simulink model "IEEE14_case"  (R2024b)
settings: Solver=FixedStepAuto  StartTime=0  StopTime=2  FixedStep=1e-7  RelTol=1e-3
values from neighbouring files (symbols this model uses):
  GFL_15_Bva = 0.009    [IEEE14_parameters.m]
  GFL_15_C_bus_pu = 7.179419    [IEEE14_parameters.m]
  GFL_15_f0 = 60    [IEEE14_parameters.m]
  GFL_15_I_id = 691.26967    [IEEE14_parameters.m]
  GFL_15_I_iq = 691.26967    [IEEE14_parameters.m]
  GFL_15_I_od = 45.2207    [IEEE14_parameters.m]
  GFL_15_I_oq = 45.2207    [IEEE14_parameters.m]
  GFL_15_I_pll = 0.78    [IEEE14_parameters.m]
  GFL_15_Kdi = 0.09    [IEEE14_parameters.m]
  GFL_15_Kdo = 0.9    [IEEE14_parameters.m]
  GFL_15_Kqi = 0.09    [IEEE14_parameters.m]
  GFL_15_Kqo = 0.9    [IEEE14_parameters.m]
  GFL_15_Lg_pu = 0.631447    [IEEE14_parameters.m]
  GFL_15_mode = 1    [IEEE14_parameters.m]
  GFL_15_P_id = 3.7166    [IEEE14_parameters.m]
  GFL_15_P_iq = 3.7166    [IEEE14_parameters.m]
  GFL_15_P_od = 0.4798    [IEEE14_parameters.m]
  GFL_15_P_oq = 0.4798    [IEEE14_parameters.m]
  GFL_15_P_pll = 290.42    [IEEE14_parameters.m]
  GFL_15_Qe_ref = 0.2    [IEEE14_parameters.m]
  GFL_15_Rg_pu = 0.024016    [IEEE14_parameters.m]
  GFL_15_Sbase = 1.000000e+4    (= 10000)    [IEEE14_parameters.m]
  GFL_15_Tdi = 0.01    [IEEE14_parameters.m]
  GFL_15_Tdo = 0.2    [IEEE14_parameters.m]
  GFL_15_Tqi = 0.01    [IEEE14_parameters.m]
  GFL_15_Tqo = 0.2    [IEEE14_parameters.m]
  GFL_15_Vbase = 380    [IEEE14_parameters.m]
  GFL_15_Vdc_ref = 1.011475    [IEEE14_parameters.m]
  GFL_15_Vdcbase = 700    [IEEE14_parameters.m]
  GFL_15_vq_ref = 0    [IEEE14_parameters.m]
  GFL_16_Bva = 0.002    [IEEE14_parameters.m]
  GFL_16_C_bus_pu = 7.179419    [IEEE14_parameters.m]
  GFL_16_f0 = 60    [IEEE14_parameters.m]
  GFL_16_I_id = 691.26967    [IEEE14_parameters.m]
  GFL_16_I_iq = 691.26967    [IEEE14_parameters.m]
  GFL_16_I_od = 45.2207    [IEEE14_parameters.m]
  GFL_16_I_oq = 45.2207    [IEEE14_parameters.m]
  GFL_16_I_pll = 0.78    [IEEE14_parameters.m]
  GFL_16_Kdi = 0.05    [IEEE14_parameters.m]
  GFL_16_Kdo = 0.5    [IEEE14_parameters.m]
  GFL_16_Kqi = 0.05    [IEEE14_parameters.m]
  GFL_16_Kqo = 0.5    [IEEE14_parameters.m]
  GFL_16_Lg_pu = 0.631447    [IEEE14_parameters.m]
  GFL_16_mode = 1    [IEEE14_parameters.m]
  GFL_16_P_id = 3.7166    [IEEE14_parameters.m]
  GFL_16_P_iq = 3.7166    [IEEE14_parameters.m]
  GFL_16_P_od = 0.4798    [IEEE14_parameters.m]
  GFL_16_P_oq = 0.4798    [IEEE14_parameters.m]
  GFL_16_P_pll = 290.42    [IEEE14_parameters.m]
  GFL_16_Qe_ref = 0.2    [IEEE14_parameters.m]
  GFL_16_Rg_pu = 0.024016    [IEEE14_parameters.m]
  GFL_16_Sbase = 1.000000e+4    (= 10000)    [IEEE14_parameters.m]
  GFL_16_Tdi = 0.01    [IEEE14_parameters.m]
  GFL_16_Tdo = 0.2    [IEEE14_parameters.m]
  GFL_16_Tqi = 0.01    [IEEE14_parameters.m]
  GFL_16_Tqo = 0.2    [IEEE14_parameters.m]
  GFL_16_Vbase = 380    [IEEE14_parameters.m]
  GFL_16_Vdc_ref = 1.01144    [IEEE14_parameters.m]
  GFL_16_Vdcbase = 700    [IEEE14_parameters.m]
  GFL_16_vq_ref = 0    [IEEE14_parameters.m]
  GFL_17_Bva = 0.002    [IEEE14_parameters.m]
  GFL_17_C_bus_pu = 7.179419    [IEEE14_parameters.m]
  GFL_17_f0 = 60    [IEEE14_parameters.m]
  GFL_17_I_id = 691.26967    [IEEE14_parameters.m]
  GFL_17_I_iq = 691.26967    [IEEE14_parameters.m]
  GFL_17_I_od = 45.2207    [IEEE14_parameters.m]
  GFL_17_I_oq = 45.2207    [IEEE14_parameters.m]
  GFL_17_I_pll = 0.78    [IEEE14_parameters.m]
  GFL_17_Kdi = 0.05    [IEEE14_parameters.m]
  GFL_17_Kdo = 0.5    [IEEE14_parameters.m]
  GFL_17_Kqi = 0.05    [IEEE14_parameters.m]
  GFL_17_Kqo = 0.5    [IEEE14_parameters.m]
  GFL_17_Lg_pu = 0.631447    [IEEE14_parameters.m]
  GFL_17_mode = 1    [IEEE14_parameters.m]
  GFL_17_P_id = 3.7166    [IEEE14_parameters.m]
  GFL_17_P_iq = 3.7166    [IEEE14_parameters.m]
  GFL_17_P_od = 0.4798    [IEEE14_parameters.m]
  GFL_17_P_oq = 0.4798    [IEEE14_parameters.m]
  GFL_17_P_pll = 290.42    [IEEE14_parameters.m]
  GFL_17_Qe_ref = 0.2    [IEEE14_parameters.m]
  GFL_17_Rg_pu = 0.024016    [IEEE14_parameters.m]
  GFL_17_Sbase = 1.000000e+4    (= 10000)    [IEEE14_parameters.m]
  GFL_17_Tdi = 0.01    [IEEE14_parameters.m]
  GFL_17_Tdo = 0.2    [IEEE14_parameters.m]
  GFL_17_Tqi = 0.01    [IEEE14_parameters.m]
  GFL_17_Tqo = 0.2    [IEEE14_parameters.m]
  GFL_17_Vbase = 380    [IEEE14_parameters.m]
  GFL_17_Vdc_ref = 1.011632    [IEEE14_parameters.m]
  GFL_17_Vdcbase = 700    [IEEE14_parameters.m]
  GFL_17_vq_ref = 0    [IEEE14_parameters.m]
  GFL_18_Bva = 0.002    [IEEE14_parameters.m]
  GFL_18_C_bus_pu = 7.179419    [IEEE14_parameters.m]
  GFL_18_f0 = 60    [IEEE14_parameters.m]
  GFL_18_I_id = 691.26967    [IEEE14_parameters.m]
  GFL_18_I_iq = 691.26967    [IEEE14_parameters.m]
  GFL_18_I_od = 45.2207    [IEEE14_parameters.m]
  GFL_18_I_oq = 45.2207    [IEEE14_parameters.m]
  GFL_18_I_pll = 0.78    [IEEE14_parameters.m]
  GFL_18_Kdi = 0.05    [IEEE14_parameters.m]
  GFL_18_Kdo = 0.5    [IEEE14_parameters.m]
  GFL_18_Kqi = 0.05    [IEEE14_parameters.m]
  GFL_18_Kqo = 0.5    [IEEE14_parameters.m]
  GFL_18_Lg_pu = 0.631447    [IEEE14_parameters.m]
  GFL_18_mode = 1    [IEEE14_parameters.m]
  GFL_18_P_id = 3.7166    [IEEE14_parameters.m]
  GFL_18_P_iq = 3.7166    [IEEE14_parameters.m]
  GFL_18_P_od = 0.4798    [IEEE14_parameters.m]
  GFL_18_P_oq = 0.4798    [IEEE14_parameters.m]
  GFL_18_P_pll = 290.42    [IEEE14_parameters.m]
  GFL_18_Qe_ref = 0.2    [IEEE14_parameters.m]
  GFL_18_Rg_pu = 0.024016    [IEEE14_parameters.m]
  GFL_18_Sbase = 1.000000e+4    (= 10000)    [IEEE14_parameters.m]
  GFL_18_Tdi = 0.01    [IEEE14_parameters.m]
  GFL_18_Tdo = 0.2    [IEEE14_parameters.m]
  GFL_18_Tqi = 0.01    [IEEE14_parameters.m]
  GFL_18_Tqo = 0.2    [IEEE14_parameters.m]
  GFL_18_Vbase = 380    [IEEE14_parameters.m]
  GFL_18_Vdc_ref = 1.011572    [IEEE14_parameters.m]
  GFL_18_Vdcbase = 700    [IEEE14_parameters.m]
  GFL_18_vq_ref = 0    [IEEE14_parameters.m]
  ... (+180 more)
(part 14 of 25)

== system IEEE14_case/GFL_18/d_Phi_gb_GFL_18_block ==
  note: d_Phi_gb_GFL_18 in case14gfl
      | $I_{\mathrm{id}}\,\left(\mathrm{Idv}_{\mathrm{GFL},18}+\Phi _{\mathrm{ga},\mathrm{GFL},18}-i_{\mathrm{gd},\mathrm{GFL},18}+P_{\mathrm{od}}\,\left(V_{\mathrm{dc},\mathrm{GFL},18}-\mathrm{Vdcbase}\,\mathrm{Vdc}_{\mathrm{ref}}\right)-\mathrm{Bva}\,\mathrm{Vbase}\,\left(v_{d,\mathrm{GFL},18}\,\cos\left(\theta _{\mathrm{pll},\mathrm{GFL},18}\right)-v_{q,\mathrm{GFL},18}\,\sin\left(\theta _{\mathrm{pll},\mathrm{GFL},18}\right)\right)\right)$
      | Automatically generated on 2025-10-09 21:37:49 .
  Input_v_d_GFL_18_d4937 : Inport
  State_theta_pll_GFL_18_76645 : Inport  Port=2
  Input_v_q_GFL_18_3c3a2 : Inport  Port=3
  State_theta_pll_GFL_18_60c54 : Inport  Port=4
  State_Idv_GFL_18_7a112 : Inport  Port=5
  State_V_dc_GFL_18_6f965 : Inport  Port=6
  State_Phi_ga_GFL_18_0803b : Inport  Port=7
  State_i_gd_GFL_18_25876 : Inport  Port=8
  Add_04fac : Sum
  Add_50ceb : Sum
  Add_6d765 : Sum
  Constant_-1_9318c : Constant  Value=-1
  Constant_Bva_df253 : Constant  Value=Bva
  Constant_I_id_6af81 : Constant  Value=I_id
  Constant_P_od_38045 : Constant  Value=P_od
  Constant_Vbase_96544 : Constant  Value=Vbase
  Constant_Vdc_ref_6e116 : Constant  Value=Vdc_ref
  Constant_Vdcbase_8f6c7 : Constant  Value=Vdcbase
  MathFunc_cos_a7f41 : Trigonometry  Operator=cos
  MathFunc_sin_0412c : Trigonometry
  Product_07db6 : Product
  Product_24552 : Product
  Product_2c113 : Product
  Product_61e81 : Product
  Product_6af82 : Product
  Product_85d52 : Product
  Product_860c9 : Product
  Product_f2f88 : Product
  Subtract_3a44e : Sum  Inputs=+-
  Subtract_78130 : Sum  Inputs=+-
  Subtract_7a8e3 : Sum  Inputs=+-
  Blockout_d_Phi_gb_GFL_18_4adfd : Outport
  wires:
  State_theta_pll_GFL_18_76645/1 -> MathFunc_cos_a7f41/1
  MathFunc_cos_a7f41/1 -> Product_61e81/2
  State_theta_pll_GFL_18_60c54/1 -> MathFunc_sin_0412c/1
  Constant_Bva_df253/1 -> Product_24552/2
  MathFunc_sin_0412c/1 -> Product_2c113/2
  Constant_-1_9318c/1 -> Product_24552/1
  State_i_gd_GFL_18_25876/1 -> Subtract_7a8e3/2
  Product_61e81/1 -> Subtract_78130/1
  Input_v_d_GFL_18_d4937/1 -> Product_61e81/1
  Input_v_q_GFL_18_3c3a2/1 -> Product_2c113/1
  Product_24552/1 -> Product_85d52/1
  Constant_Vbase_96544/1 -> Product_85d52/2
  Product_2c113/1 -> Subtract_78130/2
  Constant_I_id_6af81/1 -> Product_f2f88/1
  Product_6af82/1 -> Subtract_3a44e/2
  Constant_Vdc_ref_6e116/1 -> Product_6af82/1
  Constant_Vdcbase_8f6c7/1 -> Product_6af82/2
  State_Idv_GFL_18_7a112/1 -> Add_04fac/2
  Product_85d52/1 -> Product_07db6/1
  State_Phi_ga_GFL_18_0803b/1 -> Add_50ceb/2
  Subtract_78130/1 -> Product_07db6/2
  Subtract_3a44e/1 -> Product_860c9/2
  State_V_dc_GFL_18_6f965/1 -> Subtract_3a44e/1
  Product_07db6/1 -> Add_04fac/1
  Constant_P_od_38045/1 -> Product_860c9/1
  Add_04fac/1 -> Add_6d765/1
  Product_860c9/1 -> Add_6d765/2
  Add_6d765/1 -> Add_50ceb/1
  Add_50ceb/1 -> Subtract_7a8e3/1
  Product_f2f88/1 -> Blockout_d_Phi_gb_GFL_18_4adfd/1
  Subtract_7a8e3/1 -> Product_f2f88/2

== system IEEE14_case/GFL_18/d_Phi_gc_GFL_18_block ==
  note: d_Phi_gc_GFL_18 in case14gfl
      | $-I_{\mathrm{oq}}\,\left(\mathrm{Qe}_{\mathrm{ref}}\,\mathrm{Sbase}+1.73205080756888\,\mathrm{Vbase}\,i_{\mathrm{gd},\mathrm{GFL},18}\,\left(v_{q,\mathrm{GFL},18}\,\cos\left(\theta _{\mathrm{pll},\mathrm{GFL},18}\right)+v_{d,\mathrm{GFL},18}\,\sin\left(\theta _{\mathrm{pll},\mathrm{GFL},18}\right)\right)+1.73205080756888\,\mathrm{Vbase}\,i_{\mathrm{gq},\mathrm{GFL},18}\,\left(v_{d,\mathrm{GFL},18}\,\cos\left(\theta _{\mathrm{pll},\mathrm{GFL},18}\right)-v_{q,\mathrm{GFL},18}\,\sin\left(\theta _{\mathrm{pll},\mathrm{GFL},18}\right)\right)\right)$
      | Automatically generated on 2025-10-09 21:37:52 .
  State_i_gd_GFL_18_5899c : Inport
  Input_v_d_GFL_18_02ef3 : Inport  Port=2
  State_theta_pll_GFL_18_ce778 : Inport  Port=3
  Input_v_q_GFL_18_ef739 : Inport  Port=4
  State_theta_pll_GFL_18_3fc4b : Inport  Port=5
  State_i_gq_GFL_18_622c8 : Inport  Port=6
  Input_v_d_GFL_18_79bfc : Inport  Port=7
  State_theta_pll_GFL_18_d8932 : Inport  Port=8
  Input_v_q_GFL_18_a00d2 : Inport  Port=9
  State_theta_pll_GFL_18_57f3c : Inport  Port=10
  Add_6d69b : Sum
  Constant_-1_98670 : Constant  Value=-1
  Constant_1.73205080756888_14d38 : Constant  Value=1.73205080756888
  Constant_1.73205080756888_ac93c : Constant  Value=1.73205080756888
  Constant_I_oq_ead3f : Constant  Value=I_oq
  Constant_Qe_ref_2b81e : Constant  Value=Qe_ref
  Constant_Sbase_95d0b : Constant  Value=Sbase
  Constant_Vbase_70aa7 : Constant  Value=Vbase
  Constant_Vbase_7f599 : Constant  Value=Vbase
  MathFunc_cos_52954 : Trigonometry  Operator=cos
  MathFunc_cos_58d6c : Trigonometry  Operator=cos
  MathFunc_sin_00400 : Trigonometry
  MathFunc_sin_37ab1 : Trigonometry
  Product_0c2bb : Product
  Product_12f9b : Product
  Product_31362 : Product
  Product_3452c : Product
  Product_405b1 : Product
  Product_472e4 : Product
  Product_90b14 : Product
  Product_9a0a3 : Product
  Product_a7161 : Product
  Product_ae793 : Product
  Product_e9756 : Product
  Product_eaf4c : Product
  Product_f56c9 : Product
  Subtract_514a8 : Sum  Inputs=+-
  Subtract_9ec50 : Sum  Inputs=+-
  Subtract_a8992 : Sum  Inputs=+-
  Blockout_d_Phi_gc_GFL_18_de35a : Outport
  wires:
  State_theta_pll_GFL_18_ce778/1 -> MathFunc_sin_00400/1
  MathFunc_sin_00400/1 -> Product_9a0a3/2
  Product_f56c9/1 -> Product_ae793/1
  Constant_Qe_ref_2b81e/1 -> Product_e9756/2
  Constant_Vbase_70aa7/1 -> Product_90b14/2
  State_theta_pll_GFL_18_3fc4b/1 -> MathFunc_cos_52954/1
  Constant_1.73205080756888_14d38/1 -> Product_90b14/1
  Product_e9756/1 -> Product_3452c/1
  Constant_-1_98670/1 -> Product_e9756/1
  Input_v_d_GFL_18_02ef3/1 -> Product_9a0a3/1
  Input_v_q_GFL_18_ef739/1 -> Product_eaf4c/1
  MathFunc_cos_52954/1 -> Product_eaf4c/2
  State_theta_pll_GFL_18_d8932/1 -> MathFunc_cos_58d6c/1
  State_theta_pll_GFL_18_57f3c/1 -> MathFunc_sin_37ab1/1
  Constant_Vbase_7f599/1 -> Product_0c2bb/2
  Product_90b14/1 -> Product_31362/1
  Product_0c2bb/1 -> Product_f56c9/1
  State_i_gd_GFL_18_5899c/1 -> Product_31362/2
  Product_9a0a3/1 -> Add_6d69b/1
  Product_eaf4c/1 -> Add_6d69b/2
  Constant_1.73205080756888_ac93c/1 -> Product_0c2bb/1
  Input_v_d_GFL_18_79bfc/1 -> Product_12f9b/1
  MathFunc_cos_58d6c/1 -> Product_12f9b/2
  Product_472e4/1 -> Subtract_514a8/2
  Input_v_q_GFL_18_a00d2/1 -> Product_472e4/1
  MathFunc_sin_37ab1/1 -> Product_472e4/2
  Constant_Sbase_95d0b/1 -> Product_3452c/2
  Product_31362/1 -> Product_405b1/1
  Add_6d69b/1 -> Product_405b1/2
  Constant_I_oq_ead3f/1 -> Product_a7161/1
  State_i_gq_GFL_18_622c8/1 -> Product_f56c9/2
  Product_12f9b/1 -> Subtract_514a8/1
  Product_3452c/1 -> Subtract_9ec50/1
  Product_405b1/1 -> Subtract_9ec50/2
  Subtract_514a8/1 -> Product_ae793/2
  Product_ae793/1 -> Subtract_a8992/2
  Subtract_9ec50/1 -> Subtract_a8992/1
  Subtract_a8992/1 -> Product_a7161/2
  Product_a7161/1 -> Blockout_d_Phi_gc_GFL_18_de35a/1

== system IEEE14_case/GFL_18/d_Phi_gd_GFL_18_block ==
  note: d_Phi_gd_GFL_18 in case14gfl
      | $I_{\mathrm{iq}}\,\left(\mathrm{Iqv}_{\mathrm{GFL},18}+\Phi _{\mathrm{gc},\mathrm{GFL},18}-i_{\mathrm{gq},\mathrm{GFL},18}-P_{\mathrm{oq}}\,\left(\mathrm{Qe}_{\mathrm{ref}}\,\mathrm{Sbase}+1.73205080756888\,\mathrm{Vbase}\,i_{\mathrm{gd},\mathrm{GFL},18}\,\left(v_{q,\mathrm{GFL},18}\,\cos\left(\theta _{\mathrm{pll},\mathrm{GFL},18}\right)+v_{d,\mathrm{GFL},18}\,\sin\left(\theta _{\mathrm{pll},\mathrm{GFL},18}\right)\right)+1.73205080756888\,\mathrm{Vbase}\,i_{\mathrm{gq},\mathrm{GFL},18}\,\left(v_{d,\mathrm{GFL},18}\,\cos\left(\theta _{\mathrm{pll},\mathrm{GFL},18}\right)-v_{q,\mathrm{GFL},18}\,\sin\left(\theta _{\mathrm{pll},\mathrm{GFL},18}\right)\right)\right)+\mathrm{Bva}\,\mathrm{Vbase}\,\left(v_{q,\mathrm{GFL},18}\,\cos\left(\theta _{\mathrm{pll},\mathrm{GFL},18}\right)+v_{d,\mathrm{GFL},18}\,\sin\left(\theta _{\mathrm{pll},\mathrm{GFL},18}\right)\right)\right)$
      | Automatically generated on 2025-10-09 21:37:55 .
  Input_v_d_GFL_18_11d9f : Inport
  State_theta_pll_GFL_18_6022b : Inport  Port=2
  Input_v_q_GFL_18_3c803 : Inport  Port=3
  State_theta_pll_GFL_18_7f5d8 : Inport  Port=4
  State_Iqv_GFL_18_70c7a : Inport  Port=5
  State_i_gd_GFL_18_2dd77 : Inport  Port=6
  Input_v_d_GFL_18_27679 : Inport  Port=7
  State_theta_pll_GFL_18_40df2 : Inport  Port=8
  Input_v_q_GFL_18_95c1e : Inport  Port=9
  State_theta_pll_GFL_18_8d0fd : Inport  Port=10
  State_i_gq_GFL_18_21998 : Inport  Port=11
  Input_v_d_GFL_18_ab6ff : Inport  Port=12
  State_theta_pll_GFL_18_77a50 : Inport  Port=13
  Input_v_q_GFL_18_9cd88 : Inport  Port=14
  State_theta_pll_GFL_18_ec069 : Inport  Port=15
  State_Phi_gc_GFL_18_ff2c0 : Inport  Port=16
  State_i_gq_GFL_18_464a8 : Inport  Port=17
  Add_0e427 : Sum
  Add_719c3 : Sum
  Add_c28f7 : Sum
  Add_c4a0d : Sum
  Add_f7ea7 : Sum
  Constant_-1_1950d : Constant  Value=-1
  Constant_1.73205080756888_a5f88 : Constant  Value=1.73205080756888
  Constant_1.73205080756888_c914a : Constant  Value=1.73205080756888
  Constant_Bva_84f30 : Constant  Value=Bva
  Constant_I_iq_9a89a : Constant  Value=I_iq
  Constant_P_oq_82259 : Constant  Value=P_oq
  Constant_Qe_ref_35c82 : Constant  Value=Qe_ref
  Constant_Sbase_67118 : Constant  Value=Sbase
  Constant_Vbase_a3264 : Constant  Value=Vbase
  Constant_Vbase_c3dd2 : Constant  Value=Vbase
  Constant_Vbase_e995a : Constant  Value=Vbase
  MathFunc_cos_487b1 : Trigonometry  Operator=cos
  MathFunc_cos_b3907 : Trigonometry  Operator=cos
  MathFunc_cos_bf6e0 : Trigonometry  Operator=cos
  MathFunc_sin_7440f : Trigonometry
  MathFunc_sin_78d34 : Trigonometry
  MathFunc_sin_864f6 : Trigonometry
  Product_00030 : Product
  Product_12c61 : Product
  Product_1bd20 : Product
  Product_3073c : Product
  Product_355e6 : Product
  Product_47536 : Product
  Product_4c1e5 : Product
  Product_548e8 : Product
  Product_63936 : Product
  Product_71de5 : Product
  Product_78d03 : Product
  Product_7bf44 : Product
  Product_7d23e : Product
  Product_90c29 : Product
  Product_c3b8f : Product
  Product_f2232 : Product
  Product_f45af : Product
  Product_febba : Product
  Subtract_320f9 : Sum  Inputs=+-
  Subtract_62414 : Sum  Inputs=+-
  Subtract_8be3d : Sum  Inputs=+-
  Subtract_ed606 : Sum  Inputs=+-
  Blockout_d_Phi_gd_GFL_18_10055 : Outport
  wires:
  Product_00030/1 -> Product_12c61/1
  Constant_Vbase_c3dd2/1 -> Product_1bd20/2
  State_theta_pll_GFL_18_40df2/1 -> MathFunc_sin_7440f/1
  State_theta_pll_GFL_18_8d0fd/1 -> MathFunc_cos_487b1/1
  MathFunc_cos_487b1/1 -> Product_355e6/2
  Add_0e427/1 -> Add_c4a0d/1
  State_i_gq_GFL_18_21998/1 -> Product_00030/2
  Product_1bd20/1 -> Product_febba/1
  Constant_1.73205080756888_a5f88/1 -> Product_1bd20/1
  Constant_Vbase_e995a/1 -> Product_47536/2
  Product_548e8/1 -> Add_c28f7/1
  Constant_Qe_ref_35c82/1 -> Product_c3b8f/2
  Input_v_d_GFL_18_27679/1 -> Product_548e8/1
  Constant_Sbase_67118/1 -> Product_71de5/2
  MathFunc_sin_7440f/1 -> Product_548e8/2
  Product_355e6/1 -> Add_c28f7/2
  Input_v_q_GFL_18_95c1e/1 -> Product_355e6/1
  MathFunc_cos_bf6e0/1 -> Product_7d23e/2
  State_theta_pll_GFL_18_77a50/1 -> MathFunc_cos_bf6e0/1
  MathFunc_sin_78d34/1 -> Product_3073c/2
  State_theta_pll_GFL_18_ec069/1 -> MathFunc_sin_78d34/1
  MathFunc_sin_864f6/1 -> Product_f45af/2
  State_theta_pll_GFL_18_6022b/1 -> MathFunc_sin_864f6/1
  State_i_gq_GFL_18_464a8/1 -> Subtract_ed606/2
  MathFunc_cos_b3907/1 -> Product_7bf44/2
  State_theta_pll_GFL_18_7f5d8/1 -> MathFunc_cos_b3907/1
  Product_c3b8f/1 -> Product_71de5/1
  Constant_-1_1950d/1 -> Product_c3b8f/1
  Product_4c1e5/1 -> Product_00030/1
  Constant_1.73205080756888_c914a/1 -> Product_4c1e5/1
  State_i_gd_GFL_18_2dd77/1 -> Product_febba/2
  Product_febba/1 -> Product_90c29/1
  Constant_Vbase_a3264/1 -> Product_4c1e5/2
  Product_7d23e/1 -> Subtract_320f9/1
  Input_v_d_GFL_18_ab6ff/1 -> Product_7d23e/1
  Input_v_q_GFL_18_9cd88/1 -> Product_3073c/1
  Product_f45af/1 -> Add_719c3/1
  Input_v_d_GFL_18_11d9f/1 -> Product_f45af/1
  Input_v_q_GFL_18_3c803/1 -> Product_7bf44/1
  Add_c28f7/1 -> Product_90c29/2
  Product_3073c/1 -> Subtract_320f9/2
  Constant_Bva_84f30/1 -> Product_47536/1
  Product_7bf44/1 -> Add_719c3/2
  Product_71de5/1 -> Subtract_8be3d/1
  Product_90c29/1 -> Subtract_8be3d/2
  Subtract_320f9/1 -> Product_12c61/2
  Product_47536/1 -> Product_78d03/1
  Add_719c3/1 -> Product_78d03/2
  Add_f7ea7/1 -> Subtract_ed606/1
  Subtract_8be3d/1 -> Subtract_62414/1
  Product_12c61/1 -> Subtract_62414/2
  Product_78d03/1 -> Add_0e427/1
  Constant_I_iq_9a89a/1 -> Product_63936/1
  State_Iqv_GFL_18_70c7a/1 -> Add_0e427/2
  Constant_P_oq_82259/1 -> Product_f2232/1
  Subtract_62414/1 -> Product_f2232/2
  Product_f2232/1 -> Add_c4a0d/2
  Add_c4a0d/1 -> Add_f7ea7/1
  State_Phi_gc_GFL_18_ff2c0/1 -> Add_f7ea7/2
  Subtract_ed606/1 -> Product_63936/2
  Product_63936/1 -> Blockout_d_Phi_gd_GFL_18_10055/1

== system IEEE14_case/GFL_18/d_Phipll_GFL_18_block ==
  note: d_Phipll_GFL_18 in case14gfl
      | $-I_{\mathrm{pll}}\,\left(\mathrm{vq}_{\mathrm{ref}}+v_{q,\mathrm{GFL},18}\,\cos\left(\theta _{\mathrm{pll},\mathrm{GFL},18}\right)+v_{d,\mathrm{GFL},18}\,\sin\left(\theta _{\mathrm{pll},\mathrm{GFL},18}\right)\right)$
      | Automatically generated on 2025-10-09 21:37:46 .
  Input_v_d_GFL_18_58041 : Inport
  State_theta_pll_GFL_18_676c3 : Inport  Port=2
  Input_v_q_GFL_18_0e9bd : Inport  Port=3
  State_theta_pll_GFL_18_5129b : Inport  Port=4
  Constant_-1_3876e : Constant  Value=-1
  Constant_I_pll_a1865 : Constant  Value=I_pll
  Constant_vq_ref_f9db2 : Constant  Value=vq_ref
  MathFunc_cos_8e269 : Trigonometry  Operator=cos
  MathFunc_sin_8e406 : Trigonometry
  Product_0b2f2 : Product
  Product_65793 : Product
  Product_a3945 : Product
  Product_c4682 : Product
  Subtract_c431c : Sum  Inputs=+-
  Subtract_d6265 : Sum  Inputs=+-
  Blockout_d_Phipll_GFL_18_24764 : Outport
  wires:
  Constant_-1_3876e/1 -> Product_c4682/1
  State_theta_pll_GFL_18_5129b/1 -> MathFunc_cos_8e269/1
  Input_v_d_GFL_18_58041/1 -> Product_c4682/2
  Input_v_q_GFL_18_0e9bd/1 -> Product_65793/1
  State_theta_pll_GFL_18_676c3/1 -> MathFunc_sin_8e406/1
  MathFunc_sin_8e406/1 -> Product_0b2f2/2
  Product_c4682/1 -> Product_0b2f2/1
  MathFunc_cos_8e269/1 -> Product_65793/2
  Product_0b2f2/1 -> Subtract_c431c/1
  Product_65793/1 -> Subtract_c431c/2
  Subtract_c431c/1 -> Subtract_d6265/1
  Constant_vq_ref_f9db2/1 -> Subtract_d6265/2
  Constant_I_pll_a1865/1 -> Product_a3945/1
  Subtract_d6265/1 -> Product_a3945/2
  Product_a3945/1 -> Blockout_d_Phipll_GFL_18_24764/1

== system IEEE14_case/GFL_18/d_Psi_d_GFL_18_block ==
  note: d_Psi_d_GFL_18 in case14gfl
      | $-\frac{\Psi _{d,\mathrm{GFL},18}+\mathrm{Kdi}\,\mathrm{Vbase}\,\left(v_{q,\mathrm{GFL},18}\,\cos\left(\theta _{\mathrm{pll},\mathrm{GFL},18}\right)+v_{d,\mathrm{GFL},18}\,\sin\left(\theta _{\mathrm{pll},\mathrm{GFL},18}\right)\right)}{\mathrm{Tdi}}$
      | Automatically generated on 2025-10-09 21:37:57 .
  Input_v_d_GFL_18_5d979 : Inport
  State_theta_pll_GFL_18_3c1b0 : Inport  Port=2
  Input_v_q_GFL_18_a3318 : Inport  Port=3
  State_theta_pll_GFL_18_19ef9 : Inport  Port=4
  State_Psi_d_GFL_18_fcaf2 : Inport  Port=5
  Add_0bec6 : Sum
  Constant_-1_e13ce : Constant  Value=-1
  Constant_Kdi_70701 : Constant  Value=Kdi
  Constant_Tdi_f2ec1 : Constant  Value=Tdi
  Constant_Vbase_f17ca : Constant  Value=Vbase
  Divide_ec9ad : Product  Inputs=*/
  MathFunc_cos_215fa : Trigonometry  Operator=cos
  MathFunc_sin_1f4ca : Trigonometry
  Product_38eb0 : Product
  Product_49493 : Product
  Product_6ddec : Product
  Product_a0a46 : Product
  Product_e0f27 : Product
  Subtract_399ed : Sum  Inputs=+-
  Blockout_d_Psi_d_GFL_18_ff813 : Outport
  wires:
  MathFunc_sin_1f4ca/1 -> Product_e0f27/2
  State_Psi_d_GFL_18_fcaf2/1 -> Subtract_399ed/2
  Constant_Kdi_70701/1 -> Product_49493/2
  State_theta_pll_GFL_18_3c1b0/1 -> MathFunc_sin_1f4ca/1
  Add_0bec6/1 -> Product_6ddec/2
  State_theta_pll_GFL_18_19ef9/1 -> MathFunc_cos_215fa/1
  Input_v_q_GFL_18_a3318/1 -> Product_a0a46/1
  MathFunc_cos_215fa/1 -> Product_a0a46/2
  Constant_-1_e13ce/1 -> Product_49493/1
  Input_v_d_GFL_18_5d979/1 -> Product_e0f27/1
  Subtract_399ed/1 -> Divide_ec9ad/1
  Product_49493/1 -> Product_38eb0/1
  Constant_Vbase_f17ca/1 -> Product_38eb0/2
  Product_e0f27/1 -> Add_0bec6/1
  Product_a0a46/1 -> Add_0bec6/2
  Product_38eb0/1 -> Product_6ddec/1
  Product_6ddec/1 -> Subtract_399ed/1
  Constant_Tdi_f2ec1/1 -> Divide_ec9ad/2
  Divide_ec9ad/1 -> Blockout_d_Psi_d_GFL_18_ff813/1

== system IEEE14_case/GFL_18/d_Psi_q_GFL_18_block ==
  note: d_Psi_q_GFL_18 in case14gfl
      | $-\frac{\Psi _{q,\mathrm{GFL},18}-\mathrm{Kqi}\,\mathrm{Vbase}\,\left(v_{d,\mathrm{GFL},18}\,\cos\left(\theta _{\mathrm{pll},\mathrm{GFL},18}\right)-v_{q,\mathrm{GFL},18}\,\sin\left(\theta _{\mathrm{pll},\mathrm{GFL},18}\right)\right)}{\mathrm{Tqi}}$
      | Automatically generated on 2025-10-09 21:37:58 .
  Input_v_d_GFL_18_32a52 : Inport
  State_theta_pll_GFL_18_7c914 : Inport  Port=2
  Input_v_q_GFL_18_f7ea8 : Inport  Port=3
  State_theta_pll_GFL_18_501c5 : Inport  Port=4
  State_Psi_q_GFL_18_f8931 : Inport  Port=5
  Constant_Kqi_e65a8 : Constant  Value=Kqi
  Constant_Tqi_dc1df : Constant  Value=Tqi
  Constant_Vbase_84490 : Constant  Value=Vbase
  Divide_a8221 : Product  Inputs=*/
  MathFunc_cos_a20be : Trigonometry  Operator=cos
  MathFunc_sin_e9cc7 : Trigonometry
  Product_6e7c1 : Product
  Product_82371 : Product
  Product_c7755 : Product
  Product_ee888 : Product
  Subtract_9fd8b : Sum  Inputs=+-
  Subtract_c6d7f : Sum  Inputs=+-
  Blockout_d_Psi_q_GFL_18_327d3 : Outport
  wires:
  Product_ee888/1 -> Subtract_c6d7f/1
  Constant_Kqi_e65a8/1 -> Product_6e7c1/1
  State_theta_pll_GFL_18_7c914/1 -> MathFunc_cos_a20be/1
  MathFunc_cos_a20be/1 -> Product_82371/2
  State_theta_pll_GFL_18_501c5/1 -> MathFunc_sin_e9cc7/1
  Input_v_d_GFL_18_32a52/1 -> Product_82371/1
  Input_v_q_GFL_18_f7ea8/1 -> Product_c7755/1
  MathFunc_sin_e9cc7/1 -> Product_c7755/2
  Constant_Vbase_84490/1 -> Product_6e7c1/2
  Product_82371/1 -> Subtract_9fd8b/1
  Product_c7755/1 -> Subtract_9fd8b/2
  Product_6e7c1/1 -> Product_ee888/1
  Subtract_9fd8b/1 -> Product_ee888/2
  State_Psi_q_GFL_18_f8931/1 -> Subtract_c6d7f/2
  Subtract_c6d7f/1 -> Divide_a8221/1
  Constant_Tqi_dc1df/1 -> Divide_a8221/2
  Divide_a8221/1 -> Blockout_d_Psi_q_GFL_18_327d3/1

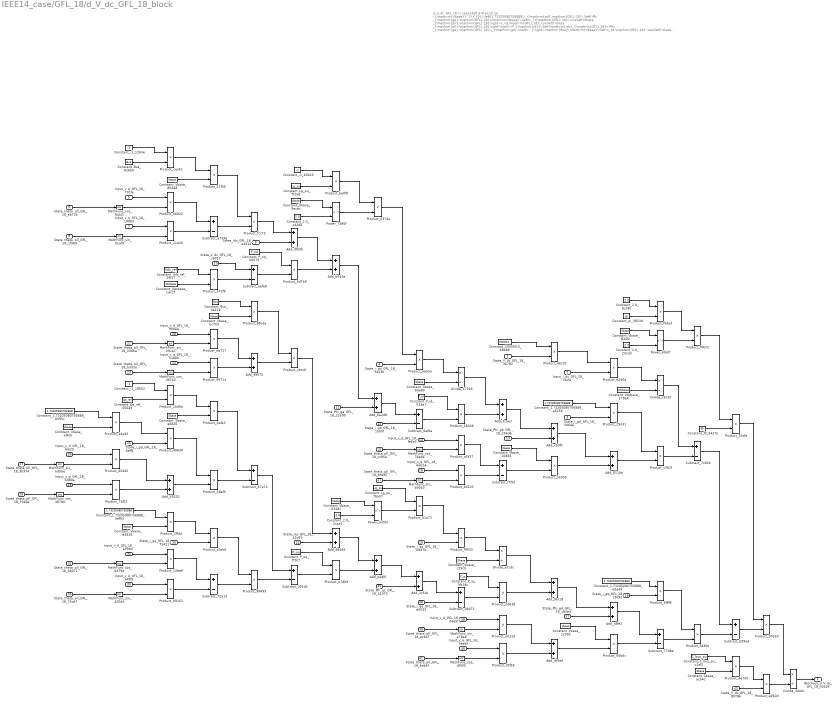
== system IEEE14_case/GFL_18/d_V_dc_GFL_18_block ==
  note: d_V_dc_GFL_18 in case14gfl
      | $-\frac{2\,\pi \,{\mathrm{Vbase}}^2\,f_{0}\,\left(1.73205080756888\,i_{\mathrm{gd},\mathrm{GFL},18}\,\left(\Phi _{\mathrm{gb},\mathrm{GFL},18}+\mathrm{Vbase}\,\left(v_{d,\mathrm{GFL},18}\,\cos\left(\theta _{\mathrm{pll},\mathrm{GFL},18}\right)-v_{q,\mathrm{GFL},18}\,\sin\left(\theta _{\mathrm{pll},\mathrm{GFL},18}\right)\right)+P_{\mathrm{id}}\,\left(\mathrm{Idv}_{\mathrm{GFL},18}+\Phi _{\mathrm{ga},\mathrm{GFL},18}-i_{\mathrm{gd},\mathrm{GFL},18}+P_{\mathrm{od}}\,\left(V_{\mathrm{dc},\mathrm{GFL},18}-\mathrm{Vdcbase}\,\mathrm{Vdc}_{\mathrm{ref}}\right)-\mathrm{Bva}\,\mathrm{Vbase}\,\left(v_{d,\mathrm{GFL},18}\,\cos\left(\theta _{\mathrm{pll},\mathrm{GFL},18}\right)-v_{q,\mathrm{GFL},18}\,\sin\left(\theta _{\mathrm{pll},\mathrm{GFL},18}\right)\right)\right)-\frac{\mathrm{Lg}_{\mathrm{pu}}\,{\mathrm{Vbase}}^2\,i_{\mathrm{gq},\mathrm{GFL},18}}{\mathrm{Sbase}}\right)+1.73205080756888\,i_{\mathrm{gq},\mathrm{GFL},18}\,\left(\Phi _{\mathrm{gd},\mathrm{GFL},18}-\mathrm{Vbase}\,\left(v_{q,\mathrm{GFL},18}\,\cos\left(\theta _{\mathrm{pll},\mathrm{GFL},18}\right)+v_{d,\mathrm{GFL},18}\,\sin\left(\theta _{\mathrm{pll},\mathrm{GFL},18}\right)\right)+P_{\mathrm{iq}}\,\left(\mathrm{Iqv}_{\mathrm{GFL},18}+\Phi _{\mathrm{gc},\mathrm{GFL},18}-i_{\mathrm{gq},\mathrm{GFL},18}-P_{\mathrm{oq}}\,\left(\mathrm{Qe}_{\mathrm{ref}}\,\mathrm{Sbase}+1.73205080756888\,\mathrm{Vbase}\,i_{\mathrm{gd},\mathrm{GFL},18}\,\left(v_{q,\mathrm{GFL},18}\,\cos\left(\theta _{\mathrm{pll},\mathrm{GFL},18}\right)+v_{d,\mathrm{GFL},18}\,\sin\left(\theta _{\mathrm{pll},\mathrm{GFL},18}\right)\right)+1.73205080756888\,\mathrm{Vbase}\,i_{\mathrm{gq},\mathrm{GFL},18}\,\left(v_{d,\mathrm{GFL},18}\,\cos\left(\theta _{\mathrm{pll},\mathrm{GFL},18}\right)-v_{q,\mathrm{GFL},18}\,\sin\left(\theta _{\mathrm{pll},\mathrm{GFL},18}\right)\right)\right)+\mathrm{Bva}\,\mathrm{Vbase}\,\left(v_{q,\mathrm{GFL},18}\,\cos\left(\theta _{\mathrm{pll},\mathrm{GFL},18}\right)+v_{d,\mathrm{GFL},18}\,\sin\left(\theta _{\mathrm{pll},\mathrm{GFL},18}\right)\right)\right)+\frac{\mathrm{Lg}_{\mathrm{pu}}\,{\mathrm{Vbase}}^2\,i_{\mathrm{gd},\mathrm{GFL},18}}{\mathrm{Sbase}}\right)-\frac{100000.0\,V_{\mathrm{dc},\mathrm{GFL},18}\,i_{\mathrm{dc},\mathrm{GFL},18}}{\mathrm{Vdcbase}}\right)}{C_{\mathrm{bus},\mathrm{pu}}\,\mathrm{Sbase}\,V_{\mathrm{dc},\mathrm{GFL},18}}$
      | Automatically generated on 2025-10-09 21:37:43 .
  State_V_dc_GFL_18_3e782 : Inport
  Input_i_dc_GFL_18_c4cfa : Inport  Port=2
  State_i_gd_GFL_18_3d6da : Inport  Port=3
  State_i_gq_GFL_18_6e18c : Inport  Port=4
  Input_v_d_GFL_18_701fe : Inport  Port=5
  State_theta_pll_GFL_18_eb734 : Inport  Port=6
  Input_v_q_GFL_18_19803 : Inport  Port=7
  State_theta_pll_GFL_18_1f369 : Inport  Port=8
  State_Idv_GFL_18_a431e : Inport  Port=9
  State_V_dc_GFL_18_c6017 : Inport  Port=10
  State_Phi_ga_GFL_18_22e90 : Inport  Port=11
  State_i_gd_GFL_18_1b00f : Inport  Port=12
  State_Phi_gb_GFL_18_256d6 : Inport  Port=13
  Input_v_d_GFL_18_fe6e3 : Inport  Port=14
  State_theta_pll_GFL_18_cc95e : Inport  Port=15
  Input_v_q_GFL_18_6eb24 : Inport  Port=16
  State_theta_pll_GFL_18_69e87 : Inport  Port=17
  State_i_gq_GFL_18_13b92 : Inport  Port=18
  State_i_gd_GFL_18_b4d7b : Inport  Port=19
  Input_v_d_GFL_18_90dae : Inport  Port=20
  State_theta_pll_GFL_18_03dba : Inport  Port=21
  Input_v_q_GFL_18_518eb : Inport  Port=22
  State_theta_pll_GFL_18_b331e : Inport  Port=23
  State_Iqv_GFL_18_42d53 : Inport  Port=24
  State_i_gd_GFL_18_beff4 : Inport  Port=25
  Input_v_d_GFL_18_feb25 : Inport  Port=26
  State_theta_pll_GFL_18_9b374 : Inport  Port=27
  Input_v_q_GFL_18_6d8da : Inport  Port=28
  State_theta_pll_GFL_18_70e0e : Inport  Port=29
  State_i_gq_GFL_18_75421 : Inport  Port=30
  Input_v_d_GFL_18_a399d : Inport  Port=31
  State_theta_pll_GFL_18_bb071 : Inport  Port=32
  Input_v_q_GFL_18_349f9 : Inport  Port=33
  State_theta_pll_GFL_18_74cd7 : Inport  Port=34
  State_Phi_gc_GFL_18_41070 : Inport  Port=35
  State_i_gq_GFL_18_e5033 : Inport  Port=36
  State_Phi_gd_GFL_18_c93e4 : Inport  Port=37
  Input_v_d_GFL_18_04e5f : Inport  Port=38
  State_theta_pll_GFL_18_ec64f : Inport  Port=39
  Input_v_q_GFL_18_9eebf : Inport  Port=40
  State_theta_pll_GFL_18_6eb5f : Inport  Port=41
  State_V_dc_GFL_18_89786 : Inport  Port=42
  Add_2c5cb : Sum
  Add_3fd3b : Sum
  Add_49232 : Sum
  Add_6a2d8 : Sum
  Add_7cae7 : Sum
  Add_811ba : Sum
  Add_98075 : Sum
  Add_9bcc8 : Sum
  Add_b4df0 : Sum
  Add_b543e : Sum
  Add_c50fb : Sum
  Add_c8fe2 : Sum
  Add_d0bef : Sum
  Add_d846d : Sum
  Constant_-1_1263e : Constant  Value=-1
  Constant_-1_18552 : Constant  Value=-1
  Constant_-1_63b25 : Constant  Value=-1
  Constant_1.73205080756888_0ef93 : Constant  Value=1.73205080756888
  Constant_1.73205080756888_8395c : Constant  Value=1.73205080756888
  Constant_1.73205080756888_a625b : Constant  Value=1.73205080756888
  Constant_1.73205080756888_e5ed6 : Constant  Value=1.73205080756888
  Constant_100000.0_48688 : Constant  Value=100000.0
  Constant_2.0_23cdd : Constant  Value=2.0
  Constant_2.0_2caa1 : Constant  Value=2.0
  Constant_2.0_8c38c : Constant  Value=2.0
  Constant_2.0_c428b : Constant  Value=2.0
  Constant_Bva_3e21e : Constant  Value=Bva
  Constant_Bva_826b6 : Constant  Value=Bva
  Constant_C_bus_pu_c1af2 : Constant  Value=C_bus_pu
  Constant_Lg_pu_76a57 : Constant  Value=Lg_pu
  Constant_Lg_pu_7f25d : Constant  Value=Lg_pu
  Constant_P_id_534e7 : Constant  Value=P_id
  Constant_P_iq_bb1dc : Constant  Value=P_iq
  Constant_P_od_bb570 : Constant  Value=P_od
  Constant_P_oq_f79c7 : Constant  Value=P_oq
  Constant_Qe_ref_656a9 : Constant  Value=Qe_ref
  Constant_Sbase_9de80 : Constant  Value=Sbase
  Constant_Sbase_acb4c : Constant  Value=Sbase
  Constant_Sbase_c19c5 : Constant  Value=Sbase
  Constant_Sbase_e6820 : Constant  Value=Sbase
  Constant_Vbase_1088d : Constant  Value=Vbase
  Constant_Vbase_2c99b : Constant  Value=Vbase
  Constant_Vbase_6328c : Constant  Value=Vbase
  Constant_Vbase_803a8 : Constant  Value=Vbase
  Constant_Vbase_9ecec : Constant  Value=Vbase
  Constant_Vbase_bc7b3 : Constant  Value=Vbase
  Constant_Vbase_e4928 : Constant  Value=Vbase
  Constant_Vbase_ef4cb : Constant  Value=Vbase
  Constant_Vbase_f4b00 : Constant  Value=Vbase
  Constant_Vdc_ref_29f17 : Constant  Value=Vdc_ref
  Constant_Vdcbase_1dcc7 : Constant  Value=Vdcbase
  Constant_Vdcbase_279e4 : Constant  Value=Vdcbase
  Constant_f0_9427b : Constant  Value=f0
  Constant_pi_3813d : Constant  Value=pi
  Divide_34a6c : Product  Inputs=*/
  Divide_47326 : Product  Inputs=*/
  Divide_c6c35 : Product  Inputs=*/
  Divide_e7cdc : Product  Inputs=*/
  MathFunc_cos_0d79d : Trigonometry  Operator=cos
  MathFunc_cos_38780 : Trigonometry  Operator=cos
  MathFunc_cos_78a8a : Trigonometry  Operator=cos
  MathFunc_cos_d9742 : Trigonometry  Operator=cos
  MathFunc_cos_df000 : Trigonometry  Operator=cos
  MathFunc_cos_f4441 : Trigonometry  Operator=cos
  MathFunc_sin_01af9 : Trigonometry
  MathFunc_sin_29c4c : Trigonometry
  MathFunc_sin_420d4 : Trigonometry
  MathFunc_sin_a78ea : Trigonometry
  MathFunc_sin_ad9ae : Trigonometry
  MathFunc_sin_b9040 : Trigonometry
  Power_535f3 : Math  Operator=pow
  Power_6fdd7 : Math  Operator=pow
  Power_7380f : Math  Operator=pow
  Product_037da : Product
  Product_05dd5 : Product
  Product_09161 : Product
  Product_{18036,21420,30350,40834,66822,96714,98499} (7 alike) : Product
  Product_1da30 : Product
  Product_21f36 : Product
  Product_24ee9 : Product
  Product_28af3 : Product
  Product_29d31 : Product
  Product_2ad8a : Product
  Product_2d638 : Product
  Product_2ff4d : Product
  Product_30f56 : Product
  Product_4af43 : Product
  Product_4d133 : Product
  Product_4e700 : Product
  Product_4ec92 : Product
  Product_54cfe : Product
  Product_5d7b9 : Product
  Product_61a72 : Product
  Product_6680c : Product
  Product_6f8f6 : Product
  Product_7bf21 : Product
  Product_85bdc : Product
  Product_88cde : Product
  Product_a060d : Product
  Product_a73f9 : Product
  Product_ba005 : Product
  Product_bd12d : Product
  Product_be0f8 : Product
  Product_c2eb6 : Product
  Product_c3b2f : Product
  Product_c6937 : Product
  Product_cbcc8 : Product
  Product_cec42 : Product
  Product_e2d0a : Product
  Product_e78b9 : Product
  Product_ee717 : Product
  Product_eea5a : Product
  Product_f4672 : Product
  Product_f5da3 : Product
  Product_f9915 : Product
  Product_fcc75 : Product
  Subtract_091d0 : Sum  Inputs=+-
  Subtract_0b071 : Sum  Inputs=+-
  Subtract_67e72 : Sum  Inputs=+-
  Subtract_6afda : Sum  Inputs=+-
  Subtract_72a13 : Sum  Inputs=+-
  Subtract_77d8e : Sum  Inputs=+-
  Subtract_7c82b : Sum  Inputs=+-
  Subtract_b99ad : Sum  Inputs=+-
  Subtract_e739e : Sum  Inputs=+-
  Subtract_eefe8 : Sum  Inputs=+-
  Subtract_f7f0d : Sum  Inputs=+-
  Blockout_d_V_dc_GFL_18_00405 : Outport
  wires:
  MathFunc_sin_ad9ae/1 -> Product_05dd5/2
  Constant_Vbase_9ecec/1 -> Power_7380f/1
  Constant_Sbase_acb4c/1 -> Product_4e700/2
  Product_6680c/1 -> Subtract_b99ad/2
  Product_2ff4d/1 -> Product_c2eb6/1
  Constant_C_bus_pu_c1af2/1 -> Product_4e700/1
  Product_54cfe/1 -> Product_30350/1
  Product_2d638/1 -> Add_9bcc8/2
  MathFunc_cos_38780/1 -> Product_7bf21/2
  Divide_34a6c/1 -> Blockout_d_V_dc_GFL_18_00405/1
  Product_a73f9/1 -> Subtract_eefe8/2
  State_V_dc_GFL_18_89786/1 -> Product_a060d/2
  Product_05dd5/1 -> Add_49232/1
  Product_29d31/1 -> Product_c3b2f/1
  Constant_Sbase_e6820/1 -> Product_4af43/2
  Product_a060d/1 -> Divide_34a6c/2
  State_i_gd_GFL_18_1b00f/1 -> Subtract_6afda/2
  Subtract_b99ad/1 -> Product_30350/2
  Constant_f0_9427b/1 -> Product_54cfe/2
  State_i_gq_GFL_18_e5033/1 -> Subtract_0b071/2
  State_theta_pll_GFL_18_b331e/1 -> MathFunc_cos_d9742/1
  Product_4e700/1 -> Product_a060d/1
  Product_fcc75/1 -> Add_3fd3b/1
  Product_30350/1 -> Divide_34a6c/1
  MathFunc_cos_0d79d/1 -> Product_24ee9/2
  Add_9bcc8/1 -> Add_c8fe2/1
  Subtract_72a13/1 -> Product_98499/2
  State_Phi_gc_GFL_18_41070/1 -> Add_2c5cb/2
  Subtract_77d8e/1 -> Product_6680c/2
  Constant_1.73205080756888_8395c/1 -> Product_1da30/1
  Divide_47326/1 -> Add_7cae7/1
  Product_2ad8a/1 -> Product_4af43/1
  Add_2c5cb/1 -> Subtract_0b071/1
  Constant_Vbase_2c99b/1 -> Product_85bdc/1
  Product_85bdc/1 -> Subtract_77d8e/2
  Subtract_6afda/1 -> Product_18036/2
  Input_v_q_GFL_18_349f9/1 -> Product_09161/1
  Product_09161/1 -> Subtract_72a13/2
  Add_b4df0/1 -> Add_2c5cb/1
  Add_d0bef/1 -> Product_85bdc/2
  Product_bd12d/1 -> Add_d0bef/1
  Subtract_f7f0d/1 -> Product_ba005/2
  Input_v_d_GFL_18_feb25/1 -> Product_05dd5/1
  Input_v_q_GFL_18_9eebf/1 -> Product_30f56/1
  Input_v_q_GFL_18_19803/1 -> Product_21420/1
  Product_30f56/1 -> Add_d0bef/2
  Subtract_0b071/1 -> Product_2d638/2
  MathFunc_cos_df000/1 -> Product_30f56/2
  State_Iqv_GFL_18_42d53/1 -> Add_d846d/2
  Product_28af3/1 -> Subtract_67e72/2
  Subtract_e739e/1 -> Product_fcc75/2
  State_theta_pll_GFL_18_6eb5f/1 -> MathFunc_cos_df000/1
  MathFunc_sin_a78ea/1 -> Product_bd12d/2
  Product_24ee9/1 -> Subtract_72a13/1
  Input_v_d_GFL_18_a399d/1 -> Product_24ee9/1
  Add_c8fe2/1 -> Subtract_77d8e/1
  Product_e78b9/1 -> Add_b4df0/2
  Product_be0f8/1 -> Product_037da/1
  Constant_Vbase_803a8/1 -> Product_21f36/2
  State_theta_pll_GFL_18_ec64f/1 -> MathFunc_sin_a78ea/1
  Constant_pi_3813d/1 -> Product_f5da3/2
  Input_v_d_GFL_18_04e5f/1 -> Product_bd12d/1
  Product_c2eb6/1 -> Product_98499/1
  State_Phi_gd_GFL_18_c93e4/1 -> Add_c8fe2/2
  Product_4af43/1 -> Subtract_67e72/1
  Constant_Sbase_9de80/1 -> Divide_47326/2
  Subtract_67e72/1 -> Subtract_091d0/1
  State_i_gd_GFL_18_b4d7b/1 -> Product_f9915/2
  Subtract_091d0/1 -> Product_e78b9/2
  Product_98499/1 -> Subtract_091d0/2
  Input_v_q_GFL_18_6d8da/1 -> Product_7bf21/1
  Product_7bf21/1 -> Add_49232/2
  Input_v_q_GFL_18_6eb24/1 -> Product_4d133/1
  State_theta_pll_GFL_18_74cd7/1 -> MathFunc_sin_420d4/1
  MathFunc_sin_420d4/1 -> Product_09161/2
  Add_49232/1 -> Product_28af3/2
  Add_811ba/1 -> Product_c3b2f/2
  Constant_Vbase_ef4cb/1 -> Product_1da30/2
  State_theta_pll_GFL_18_bb071/1 -> MathFunc_cos_0d79d/1
  State_i_gq_GFL_18_75421/1 -> Product_c2eb6/2
  Constant_Vbase_e4928/1 -> Product_2ff4d/2
  State_theta_pll_GFL_18_9b374/1 -> MathFunc_sin_ad9ae/1
  Constant_1.73205080756888_0ef93/1 -> Product_2ff4d/1
  State_theta_pll_GFL_18_70e0e/1 -> MathFunc_cos_38780/1
  Product_40834/1 -> Product_28af3/1
  Product_c3b2f/1 -> Subtract_7c82b/2
  Constant_Sbase_c19c5/1 -> Divide_e7cdc/2
  MathFunc_cos_f4441/1 -> Product_66822/2
  Add_c50fb/1 -> Add_811ba/1
  State_i_gd_GFL_18_beff4/1 -> Product_40834/2
  Product_1da30/1 -> Product_40834/1
  Constant_Qe_ref_656a9/1 -> Product_2ad8a/2
  Constant_-1_18552/1 -> Product_2ad8a/1
  MathFunc_cos_d9742/1 -> Product_96714/2
  State_i_gq_GFL_18_6e18c/1 -> Product_eea5a/2
  Constant_P_oq_f79c7/1 -> Product_e78b9/1
  Add_d846d/1 -> Add_b4df0/1
  Subtract_7c82b/1 -> Subtract_b99ad/1
  Constant_-1_63b25/1 -> Product_be0f8/1
  Product_cbcc8/1 -> Add_d846d/1
  Add_98075/1 -> Product_cbcc8/2
  Product_96714/1 -> Add_98075/2
  Input_v_q_GFL_18_518eb/1 -> Product_96714/1
  MathFunc_sin_29c4c/1 -> Product_ee717/2
  State_i_gd_GFL_18_3d6da/1 -> Product_29d31/2
  Product_ee717/1 -> Add_98075/1
  State_theta_pll_GFL_18_03dba/1 -> MathFunc_sin_29c4c/1
  Input_v_d_GFL_18_90dae/1 -> Product_ee717/1
  Product_88cde/1 -> Product_cbcc8/1
  Constant_Vbase_bc7b3/1 -> Product_88cde/2
  Constant_Bva_3e21e/1 -> Product_88cde/1
  Constant_P_iq_bb1dc/1 -> Product_2d638/1
  State_V_dc_GFL_18_3e782/1 -> Product_4ec92/2
  Divide_e7cdc/1 -> Add_9bcc8/1
  Product_f9915/1 -> Divide_e7cdc/1
  Product_61a72/1 -> Product_f9915/1
  Power_535f3/1 -> Product_61a72/2
  Constant_2.0_2caa1/1 -> Power_535f3/2
  Constant_Vbase_6328c/1 -> Power_535f3/1
  Constant_Lg_pu_76a57/1 -> Product_61a72/1
  Product_6f8f6/1 -> Product_6680c/1
  State_i_gq_GFL_18_13b92/1 -> Product_6f8f6/2
  Constant_1.73205080756888_e5ed6/1 -> Product_6f8f6/1
  Product_ba005/1 -> Add_811ba/2
  Product_4d133/1 -> Subtract_f7f0d/2
  MathFunc_sin_b9040/1 -> Product_4d133/2
  State_theta_pll_GFL_18_69e87/1 -> MathFunc_sin_b9040/1
  Product_c6937/1 -> Subtract_f7f0d/1
  MathFunc_cos_78a8a/1 -> Product_c6937/2
  State_theta_pll_GFL_18_cc95e/1 -> MathFunc_cos_78a8a/1
  Input_v_d_GFL_18_fe6e3/1 -> Product_c6937/1
  Constant_Vbase_1088d/1 -> Product_ba005/1
  State_theta_pll_GFL_18_eb734/1 -> MathFunc_cos_f4441/1
  State_Phi_gb_GFL_18_256d6/1 -> Add_c50fb/2
  Constant_P_od_bb570/1 -> Product_5d7b9/1
  Add_7cae7/1 -> Add_c50fb/1
  Product_18036/1 -> Add_7cae7/2
  Add_6a2d8/1 -> Subtract_6afda/1
  State_Phi_ga_GFL_18_22e90/1 -> Add_6a2d8/2
  Constant_Vdcbase_279e4/1 -> Divide_c6c35/2
  Add_b543e/1 -> Add_6a2d8/1
  Power_7380f/1 -> Product_037da/2
  Product_5d7b9/1 -> Add_b543e/2
  State_Idv_GFL_18_a431e/1 -> Add_3fd3b/2
  Subtract_eefe8/1 -> Product_5d7b9/2
  Constant_Vdcbase_1dcc7/1 -> Product_a73f9/2
  Constant_Vdc_ref_29f17/1 -> Product_a73f9/1
  State_V_dc_GFL_18_c6017/1 -> Subtract_eefe8/1
  Add_3fd3b/1 -> Add_b543e/1
  Constant_2.0_23cdd/1 -> Power_6fdd7/2
  Product_21420/1 -> Subtract_e739e/2
  MathFunc_sin_01af9/1 -> Product_21420/2
  State_theta_pll_GFL_18_1f369/1 -> MathFunc_sin_01af9/1
  Product_66822/1 -> Subtract_e739e/1
  Input_v_d_GFL_18_701fe/1 -> Product_66822/1
  Product_21f36/1 -> Product_fcc75/1
  Product_cec42/1 -> Product_21f36/1
  Constant_Bva_826b6/1 -> Product_cec42/2
  Constant_-1_1263e/1 -> Product_cec42/1
  Product_f5da3/1 -> Product_f4672/1
  Constant_P_id_534e7/1 -> Product_18036/1
  Product_eea5a/1 -> Divide_47326/1
  Input_i_dc_GFL_18_c4cfa/1 -> Product_e2d0a/2
  Product_037da/1 -> Product_eea5a/1
  Constant_2.0_c428b/1 -> Power_7380f/2
  Constant_Lg_pu_7f25d/1 -> Product_be0f8/2
  Constant_1.73205080756888_a625b/1 -> Product_29d31/1
  Divide_c6c35/1 -> Subtract_7c82b/1
  Product_e2d0a/1 -> Divide_c6c35/1
  Product_4ec92/1 -> Product_e2d0a/1
  Constant_100000.0_48688/1 -> Product_4ec92/1
  Product_f4672/1 -> Product_54cfe/1
  Power_6fdd7/1 -> Product_f4672/2
  Constant_Vbase_f4b00/1 -> Power_6fdd7/1
  Constant_2.0_8c38c/1 -> Product_f5da3/1

== system IEEE14_case/GFL_18/d_i_gd_GFL_18_block ==
  note: d_i_gd_GFL_18 in case14gfl
      | $\frac{2\,\pi \,\mathrm{Sbase}\,f_{0}\,\left(\Phi _{\mathrm{gb},\mathrm{GFL},18}+P_{\mathrm{id}}\,\left(\mathrm{Idv}_{\mathrm{GFL},18}+\Phi _{\mathrm{ga},\mathrm{GFL},18}-i_{\mathrm{gd},\mathrm{GFL},18}+P_{\mathrm{od}}\,\left(V_{\mathrm{dc},\mathrm{GFL},18}-\mathrm{Vdcbase}\,\mathrm{Vdc}_{\mathrm{ref}}\right)-\mathrm{Bva}\,\mathrm{Vbase}\,\left(v_{d,\mathrm{GFL},18}\,\cos\left(\theta _{\mathrm{pll},\mathrm{GFL},18}\right)-v_{q,\mathrm{GFL},18}\,\sin\left(\theta _{\mathrm{pll},\mathrm{GFL},18}\right)\right)\right)-\frac{\mathrm{Rg}_{\mathrm{pu}}\,{\mathrm{Vbase}}^2\,i_{\mathrm{gd},\mathrm{GFL},18}}{\mathrm{Sbase}}\right)}{\mathrm{Lg}_{\mathrm{pu}}\,{\mathrm{Vbase}}^2}$
      | Automatically generated on 2025-10-09 21:37:26 .
  Input_v_d_GFL_18_95c19 : Inport
  State_theta_pll_GFL_18_c6cb4 : Inport  Port=2
  Input_v_q_GFL_18_169b9 : Inport  Port=3
  State_theta_pll_GFL_18_bdc92 : Inport  Port=4
  State_Idv_GFL_18_f8d07 : Inport  Port=5
  State_V_dc_GFL_18_90391 : Inport  Port=6
  State_Phi_ga_GFL_18_805dd : Inport  Port=7
  State_i_gd_GFL_18_d4705 : Inport  Port=8
  State_Phi_gb_GFL_18_e630d : Inport  Port=9
  State_i_gd_GFL_18_ac69d : Inport  Port=10
  Add_1e609 : Sum
  Add_31210 : Sum
  Add_625ec : Sum
  Add_acf3f : Sum
  Constant_-1_da123 : Constant  Value=-1
  Constant_2.0_64485 : Constant  Value=2.0
  Constant_2.0_d7fba : Constant  Value=2.0
  Constant_2.0_f01e0 : Constant  Value=2.0
  Constant_Bva_85260 : Constant  Value=Bva
  Constant_Lg_pu_6f139 : Constant  Value=Lg_pu
  Constant_P_id_2e36a : Constant  Value=P_id
  Constant_P_od_fe442 : Constant  Value=P_od
  Constant_Rg_pu_dad66 : Constant  Value=Rg_pu
  Constant_Sbase_1c6cd : Constant  Value=Sbase
  Constant_Sbase_ab842 : Constant  Value=Sbase
  Constant_Vbase_0fc7d : Constant  Value=Vbase
  Constant_Vbase_521dd : Constant  Value=Vbase
  Constant_Vbase_8420d : Constant  Value=Vbase
  Constant_Vdc_ref_7b8c6 : Constant  Value=Vdc_ref
  Constant_Vdcbase_e67af : Constant  Value=Vdcbase
  Constant_f0_3d1cd : Constant  Value=f0
  Constant_pi_7e6bc : Constant  Value=pi
  Divide_6844e : Product  Inputs=*/
  Divide_7e982 : Product  Inputs=*/
  MathFunc_cos_d65d0 : Trigonometry  Operator=cos
  MathFunc_sin_305f9 : Trigonometry
  Power_53e10 : Math  Operator=pow
  Power_cd5de : Math  Operator=pow
  Product_054e5 : Product
  Product_0613f : Product
  Product_1e093 : Product
  Product_2a8fd : Product
  Product_2d7e3 : Product
  Product_54c77 : Product
  Product_5eb62 : Product
  Product_6d394 : Product
  Product_70042 : Product
  Product_9298c : Product
  Product_984f3 : Product
  Product_b28c9 : Product
  Product_d4748 : Product
  Product_ebe76 : Product
  Product_f53c4 : Product
  Subtract_03e05 : Sum  Inputs=+-
  Subtract_6c6cd : Sum  Inputs=+-
  Subtract_7b94e : Sum  Inputs=+-
  Subtract_f1451 : Sum  Inputs=+-
  Blockout_d_i_gd_GFL_18_28d76 : Outport
  wires:
  State_theta_pll_GFL_18_c6cb4/1 -> MathFunc_cos_d65d0/1
  MathFunc_cos_d65d0/1 -> Product_d4748/2
  Product_984f3/1 -> Add_31210/2
  Constant_Bva_85260/1 -> Product_f53c4/2
  State_theta_pll_GFL_18_bdc92/1 -> MathFunc_sin_305f9/1
  MathFunc_sin_305f9/1 -> Product_5eb62/2
  Constant_-1_da123/1 -> Product_f53c4/1
  Product_d4748/1 -> Subtract_f1451/1
  Input_v_d_GFL_18_95c19/1 -> Product_d4748/1
  Input_v_q_GFL_18_169b9/1 -> Product_5eb62/1
  Product_f53c4/1 -> Product_054e5/1
  Constant_P_od_fe442/1 -> Product_984f3/1
  Constant_Vbase_521dd/1 -> Product_054e5/2
  Product_5eb62/1 -> Subtract_f1451/2
  Product_54c77/1 -> Divide_6844e/1
  Product_9298c/1 -> Subtract_03e05/2
  Constant_Vdc_ref_7b8c6/1 -> Product_9298c/1
  Power_cd5de/1 -> Product_0613f/2
  Constant_Vdcbase_e67af/1 -> Product_9298c/2
  Product_054e5/1 -> Product_70042/1
  Subtract_f1451/1 -> Product_70042/2
  Subtract_03e05/1 -> Product_984f3/2
  State_V_dc_GFL_18_90391/1 -> Subtract_03e05/1
  Constant_Sbase_1c6cd/1 -> Product_2d7e3/2
  Product_70042/1 -> Add_625ec/1
  State_Idv_GFL_18_f8d07/1 -> Add_625ec/2
  Constant_pi_7e6bc/1 -> Product_6d394/2
  Add_625ec/1 -> Add_31210/1
  Add_31210/1 -> Add_acf3f/1
  Product_0613f/1 -> Product_b28c9/1
  State_Phi_ga_GFL_18_805dd/1 -> Add_acf3f/2
  Constant_2.0_f01e0/1 -> Power_cd5de/2
  Constant_Vbase_8420d/1 -> Power_cd5de/1
  Constant_f0_3d1cd/1 -> Product_ebe76/2
  Add_acf3f/1 -> Subtract_7b94e/1
  State_i_gd_GFL_18_d4705/1 -> Subtract_7b94e/2
  Constant_Rg_pu_dad66/1 -> Product_0613f/1
  Product_6d394/1 -> Product_2d7e3/1
  Constant_2.0_d7fba/1 -> Product_6d394/1
  Constant_P_id_2e36a/1 -> Product_1e093/1
  Subtract_7b94e/1 -> Product_1e093/2
  State_i_gd_GFL_18_ac69d/1 -> Product_b28c9/2
  Product_1e093/1 -> Add_1e609/1
  State_Phi_gb_GFL_18_e630d/1 -> Add_1e609/2
  Product_b28c9/1 -> Divide_7e982/1
  Product_ebe76/1 -> Product_54c77/1
  Constant_Sbase_ab842/1 -> Divide_7e982/2
  Product_2d7e3/1 -> Product_ebe76/1
  Add_1e609/1 -> Subtract_6c6cd/1
  Divide_7e982/1 -> Subtract_6c6cd/2
  Constant_Vbase_0fc7d/1 -> Power_53e10/1
  Constant_2.0_64485/1 -> Power_53e10/2
  Subtract_6c6cd/1 -> Product_54c77/2
  Product_2a8fd/1 -> Divide_6844e/2
  Constant_Lg_pu_6f139/1 -> Product_2a8fd/1
  Power_53e10/1 -> Product_2a8fd/2
  Divide_6844e/1 -> Blockout_d_i_gd_GFL_18_28d76/1
